simulink model "Loops1"  (Simulink 8.7)
settings: Solver=ode45  StartTime=0.0  StopTime=10.0  RelTol=1e-3
settings Model: Creator=scaife  LastModifiedBy=bourbouh  ExtModeAutoUpdateStatusClock=off
settings DataIOCC: SignalLoggingSaveFormat=ModelDataLogs  SignalLoggingName=sigsOut
settings OptimizationCC: InitFltsAndDblsToZero=on
settings DebuggingCC: SaveWithParameterizedLinksMsg=none  SignalResolutionControl=TryResolveAllWithWarning  MultiTaskDSMMsg=warning  MultiTaskCondExecSysMsg=none
settings HardwareCC: TargetUnknown=on
settings SFSimCC: SimParseCustomCode=off
settings GRTTargetCC: TargetFcnLib=ansi_tfl_tmw.mat  ModelReferenceCompliant=off  GeneratePreprocessorConditionals=Use local settings  CombineOutputUpdateFcns=off  MatFileLogging=off  GRTInterface=on

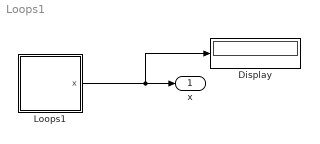
== system Loops1 ==
  Display : Display
  Loops1 : Stateflow chart  TreatAsAtomicUnit=on
  x : Outport
  wires:
  Loops1/1(x) -> Display/1, x/1

== stateflow chart Loops1 ==
  state A
  state B
  (default) -> A
  B -> A
  A -> (junction 6) : {x=0}
  (junction 6) -> (junction 6) [order 1] : [x<2]{x++}
  (junction 6) -> B [order 2]
  data: x output int32
